simulink model "quadrotor_PID_LQR_decentralized_simulink"  (R2023b)
settings: Solver=ode4  StartTime=0.0  StopTime=10  FixedStep=0.001  RelTol=1e-3
values from neighbouring files (symbols this model uses):
  A_x_in = [0 1; 0 0]    [quadrotor_PID_Hinf_Backstepping_decentralized.m]    (also in quadrotor_PID_Hinf_Synthesis_decentralized.m; quadrotor_PID_LQR_decentralized.m)
  A_x_out = [0 1; 0 0]    [quadrotor_PID_Hinf_Backstepping_decentralized.m]    (also in quadrotor_PID_Hinf_Synthesis_decentralized.m; quadrotor_PID_LQR_decentralized.m)
  A_x_pitch = [0 1  0  0 ... (first row only)    [quadrotor_PID_LQR_decentralized.m]
  A_y_in = [0 1; 0 0]    [quadrotor_PID_Hinf_Backstepping_decentralized.m]    (also in quadrotor_PID_Hinf_Synthesis_decentralized.m; quadrotor_PID_LQR_decentralized.m)
  A_y_out = [0 1; 0 0]    [quadrotor_PID_Hinf_Backstepping_decentralized.m]    (also in quadrotor_PID_Hinf_Synthesis_decentralized.m; quadrotor_PID_LQR_decentralized.m)
  A_y_roll = [0 1  0  0 ... (first row only)    [quadrotor_PID_LQR_decentralized.m]
  Ayaw = [0 1; 0 0]    [quadrotor_PID_Hinf_Backstepping_decentralized.m]    (also in quadrotor_PID_Hinf_Synthesis_decentralized.m; quadrotor_PID_LQR_decentralized.m)
  Az = [0 1; 0 0]    [quadrotor_PID_Hinf_Backstepping_decentralized.m]    (also in quadrotor_PID_Hinf_Synthesis_decentralized.m; quadrotor_PID_LQR_decentralized.m)
  B_x_in = [0; 1/Iy]    [quadrotor_PID_Hinf_Backstepping_decentralized.m]    (also in quadrotor_PID_Hinf_Synthesis_decentralized.m; quadrotor_PID_LQR_decentralized.m)
  B_x_out = [0; g]    [quadrotor_PID_Hinf_Backstepping_decentralized.m]    (also in quadrotor_PID_Hinf_Synthesis_decentralized.m; quadrotor_PID_LQR_decentralized.m)
  B_x_pitch = [0; 0; 0; 1/Iy]    [quadrotor_PID_LQR_decentralized.m]
  B_y_in = [0; 1/Ix]    [quadrotor_PID_Hinf_Backstepping_decentralized.m]    (also in quadrotor_PID_Hinf_Synthesis_decentralized.m; quadrotor_PID_LQR_decentralized.m)
  B_y_out = [0; -g]    [quadrotor_PID_Hinf_Backstepping_decentralized.m]    (also in quadrotor_PID_Hinf_Synthesis_decentralized.m; quadrotor_PID_LQR_decentralized.m)
  B_y_roll = [0; 0; 0; 1/Ix]    [quadrotor_PID_LQR_decentralized.m]
  Byaw = [0; 1/Iz]    [quadrotor_PID_Hinf_Backstepping_decentralized.m]    (also in quadrotor_PID_Hinf_Synthesis_decentralized.m; quadrotor_PID_LQR_decentralized.m)
  Bz = [0; 1/m]    [quadrotor_PID_Hinf_Backstepping_decentralized.m]    (also in quadrotor_PID_Hinf_Synthesis_decentralized.m; quadrotor_PID_LQR_decentralized.m)
  C_x_in = [1 0]    [quadrotor_PID_Hinf_Backstepping_decentralized.m]    (also in quadrotor_PID_Hinf_Synthesis_decentralized.m; quadrotor_PID_LQR_decentralized.m)
  C_x_out = [1 0]    [quadrotor_PID_Hinf_Backstepping_decentralized.m]    (also in quadrotor_PID_Hinf_Synthesis_decentralized.m; quadrotor_PID_LQR_decentralized.m)
  C_x_pitch = [1 0 0 0]    [quadrotor_PID_LQR_decentralized.m]
  C_y_in = [1 0]    [quadrotor_PID_Hinf_Backstepping_decentralized.m]    (also in quadrotor_PID_Hinf_Synthesis_decentralized.m; quadrotor_PID_LQR_decentralized.m)
  C_y_out = [1 0]    [quadrotor_PID_Hinf_Backstepping_decentralized.m]    (also in quadrotor_PID_Hinf_Synthesis_decentralized.m; quadrotor_PID_LQR_decentralized.m)
  C_y_roll = [1 0 0 0]    [quadrotor_PID_LQR_decentralized.m]
  Cyaw = [1 0]    [quadrotor_PID_Hinf_Backstepping_decentralized.m]    (also in quadrotor_PID_Hinf_Synthesis_decentralized.m; quadrotor_PID_LQR_decentralized.m)
  Cz = [1 0]    [quadrotor_PID_Hinf_Backstepping_decentralized.m]    (also in quadrotor_PID_Hinf_Synthesis_decentralized.m; quadrotor_PID_LQR_decentralized.m)
  Ku_x_pitch = K_opt_x(5)    [quadrotor_PID_LQR_decentralized.m]
  Ku_y_roll = K_opt(5)    [quadrotor_PID_LQR_decentralized.m]
  Kx_x_pitch = K_opt_x(1:4)    [quadrotor_PID_LQR_decentralized.m]
  Kx_y_roll = K_opt(1:4)    [quadrotor_PID_LQR_decentralized.m]
undefined symbols (not defined in the file or in its folder): Kd_x_in, Kd_x_out, Kd_y_in, Kd_y_out, Kd_yaw, Kd_z, Ki_x_in, Ki_x_out, Ki_y_in, Ki_y_out, Ki_yaw, Ki_z, Kp_x_in, Kp_x_out, Kp_y_in, Kp_y_out, Kp_yaw, Kp_z, Ku_yaw, Ku_z, Kx_yaw, Kx_z
libraries: dspsrcs4 x4
settings Model: Creator=izmah  LastModifiedBy=izmah

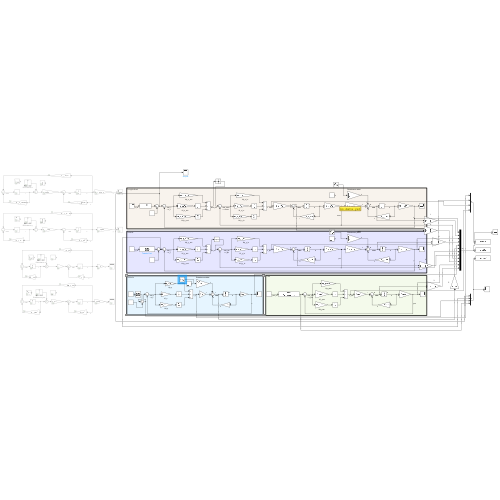
[thumbnail: Simulink's stored preview of the top-level diagram]
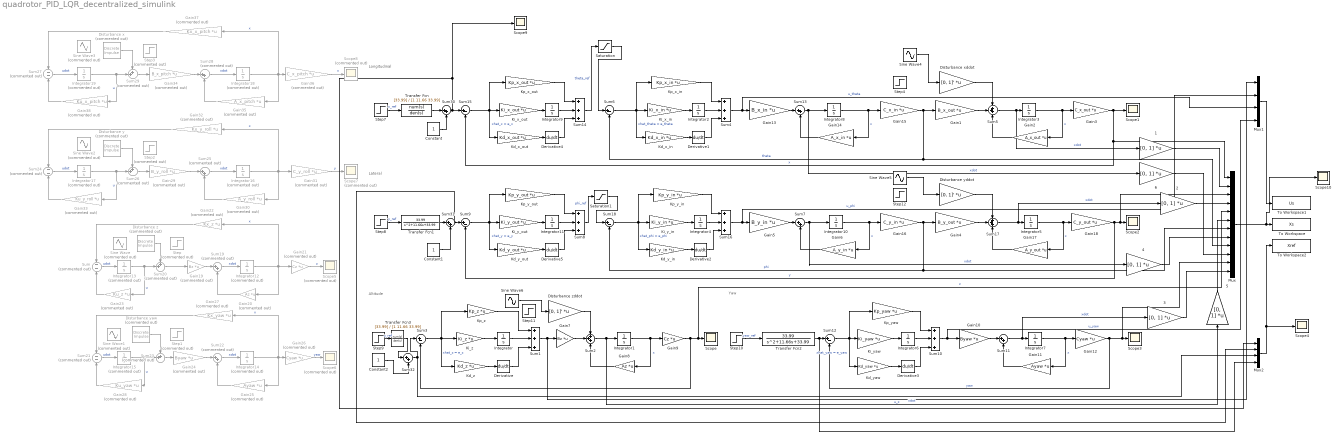
== system quadrotor_PID_LQR_decentralized_simulink ==
  note: Longitudinal
  note: Lateral
  note: Yaw
  note: Altitude
  {1..6} (6 alike) : Gain  Gain=[0, 1]  Multiplication=Matrix(K*u)
  Constant : Constant
  Constant1 : Constant
  Constant2 : Constant
  DIsturbance yddot : Gain  Gain=[0, 1]'  Multiplication=Matrix(K*u)
  DIsturbance zddot : Gain  Gain=[0, 1]'  Multiplication=Matrix(K*u)
  Derivative{,1..5} (6 alike) : Derivative
  Disturbance x : dspsrcs4/Discrete  Impulse  Commented=on  Delay=10  SampleTime=1  FrameSample=1  OutputFrames=off  dataType=double  isSigned=on  wordLen=16  udDataType=sfix(16)  fracBitsMode=Best precision  numFracBits=15  OutDataTypeStr=double  LastOutDataTypeStr=double
  Disturbance xddot : Gain  Gain=[0, 1]'  Multiplication=Matrix(K*u)
  Disturbance y : dspsrcs4/Discrete  Impulse  Commented=on  Delay=10  SampleTime=1  FrameSample=1  OutputFrames=off  dataType=double  isSigned=on  wordLen=16  udDataType=sfix(16)  fracBitsMode=Best precision  numFracBits=15  OutDataTypeStr=double  LastOutDataTypeStr=double
  Disturbance yaw : dspsrcs4/Discrete  Impulse  Commented=on  Delay=10  SampleTime=1  FrameSample=1  OutputFrames=off  dataType=double  isSigned=on  wordLen=16  udDataType=sfix(16)  fracBitsMode=Best precision  numFracBits=15  OutDataTypeStr=double  LastOutDataTypeStr=double
  Disturbance z : dspsrcs4/Discrete  Impulse  Commented=on  Delay=10  SampleTime=1  FrameSample=1  OutputFrames=off  dataType=double  isSigned=on  wordLen=16  udDataType=sfix(16)  fracBitsMode=Best precision  numFracBits=15  OutDataTypeStr=double  LastOutDataTypeStr=double
  Gain1 : Gain  Gain=B_x_out  Multiplication=Matrix(K*u)
  Gain10 : Gain  Gain=Byaw  Multiplication=Matrix(K*u)
  Gain11 : Gain  Gain=Ayaw  Multiplication=Matrix(K*u)
  Gain12 : Gain  Gain=Cyaw  Multiplication=Matrix(K*u)
  Gain13 : Gain  Gain=B_x_in  Multiplication=Matrix(K*u)
  Gain14 : Gain  Gain=A_x_in  Multiplication=Matrix(K*u)
  Gain15 : Gain  Gain=C_x_in  Multiplication=Matrix(K*u)
  Gain16 : Gain  Gain=C_y_in  Multiplication=Matrix(K*u)
  Gain17 : Gain  Gain=A_y_out  Multiplication=Matrix(K*u)
  Gain18 : Gain  Gain=C_y_out  Multiplication=Matrix(K*u)
  Gain19 : Gain  Commented=on  Gain=Bz  Multiplication=Matrix(K*u)
  Gain2 : Gain  Gain=A_x_out  Multiplication=Matrix(K*u)
  Gain20 : Gain  Commented=on  Gain=Az  Multiplication=Matrix(K*u)
  Gain21 : Gain  Commented=on  Gain=Cz  Multiplication=Matrix(K*u)
  Gain22 : Gain  Commented=on  Gain=Kx_z  Multiplication=Matrix(K*u)
  Gain23 : Gain  Commented=on  Gain=Ku_z  Multiplication=Matrix(K*u)
  Gain24 : Gain  Commented=on  Gain=Byaw  Multiplication=Matrix(K*u)
  Gain25 : Gain  Commented=on  Gain=Ayaw  Multiplication=Matrix(K*u)
  Gain26 : Gain  Commented=on  Gain=Cyaw  Multiplication=Matrix(K*u)
  Gain27 : Gain  Commented=on  Gain=Kx_yaw  Multiplication=Matrix(K*u)
  Gain28 : Gain  Commented=on  Gain=Ku_yaw  Multiplication=Matrix(K*u)
  Gain29 : Gain  Commented=on  Gain=B_y_roll  Multiplication=Matrix(K*u)
  Gain3 : Gain  Gain=C_x_out  Multiplication=Matrix(K*u)
  Gain30 : Gain  Commented=on  Gain=A_y_roll  Multiplication=Matrix(K*u)
  Gain31 : Gain  Commented=on  Gain=C_y_roll  Multiplication=Matrix(K*u)
  Gain32 : Gain  Commented=on  Gain=Kx_y_roll  Multiplication=Matrix(K*u)
  Gain33 : Gain  Commented=on  Gain=Ku_y_roll  Multiplication=Matrix(K*u)
  Gain34 : Gain  Commented=on  Gain=B_x_pitch  Multiplication=Matrix(K*u)
  Gain35 : Gain  Commented=on  Gain=A_x_pitch  Multiplication=Matrix(K*u)
  Gain36 : Gain  Commented=on  Gain=C_x_pitch  Multiplication=Matrix(K*u)
  Gain37 : Gain  Commented=on  Gain=Kx_x_pitch  Multiplication=Matrix(K*u)
  Gain38 : Gain  Commented=on  Gain=Ku_x_pitch  Multiplication=Matrix(K*u)
  Gain4 : Gain  Gain=B_y_out  Multiplication=Matrix(K*u)
  Gain5 : Gain  Gain=B_y_in  Multiplication=Matrix(K*u)
  Gain6 : Gain  Gain=A_y_in  Multiplication=Matrix(K*u)
  Gain7 : Gain  Gain=Bz  Multiplication=Matrix(K*u)
  Gain8 : Gain  Gain=Az  Multiplication=Matrix(K*u)
  Gain9 : Gain  Gain=Cz  Multiplication=Matrix(K*u)
  Integrator{,2,4,6..7,9,11} (7 alike) : Integrator
  Integrator1 : Integrator  InitialCondition=[1;0]
  Integrator10 : Integrator  InitialCondition=[0.01;0]
  Integrator{12..19} (8 alike) : Integrator  Commented=on
  Integrator3 : Integrator  InitialCondition=[1;0]
  Integrator5 : Integrator  InitialCondition=[1;0]
  Integrator8 : Integrator  InitialCondition=[0.01;0]
  Kd_x_in : Gain  Gain=Kd_x_in  Multiplication=Matrix(K*u)
  Kd_x_out : Gain  Gain=Kd_x_out  Multiplication=Matrix(K*u)
  Kd_y_in : Gain  Gain=Kd_y_in  Multiplication=Matrix(K*u)
  Kd_y_out : Gain  Gain=Kd_y_out  Multiplication=Matrix(K*u)
  Kd_yaw : Gain  Gain=Kd_yaw  Multiplication=Matrix(K*u)
  Kd_z : Gain  Gain=Kd_z  Multiplication=Matrix(K*u)
  Ki_x_in : Gain  Gain=Ki_x_in  Multiplication=Matrix(K*u)
  Ki_x_out : Gain  Gain=Ki_x_out  Multiplication=Matrix(K*u)
  Ki_y_in : Gain  Gain=Ki_y_in  Multiplication=Matrix(K*u)
  Ki_y_out : Gain  Gain=Ki_y_out  Multiplication=Matrix(K*u)
  Ki_yaw : Gain  Gain=Ki_yaw  Multiplication=Matrix(K*u)
  Ki_z : Gain  Gain=Ki_z  Multiplication=Matrix(K*u)
  Kp_x_in : Gain  Gain=Kp_x_in  Multiplication=Matrix(K*u)
  Kp_x_out : Gain  Gain=Kp_x_out  Multiplication=Matrix(K*u)
  Kp_y_in : Gain  Gain=Kp_y_in  Multiplication=Matrix(K*u)
  Kp_y_out : Gain  Gain=Kp_y_out  Multiplication=Matrix(K*u)
  Kp_yaw : Gain  Gain=Kp_yaw  Multiplication=Matrix(K*u)
  Kp_z : Gain  Gain=Kp_z  Multiplication=Matrix(K*u)
  Mux : Mux  Inputs=12
  Mux1 : Mux
  Mux2 : Mux
  Saturation : Saturate  UpperLimit=deg2rad(15)  LowerLimit=-deg2rad(15)  ZeroCross=off
  Saturation1 : Saturate  UpperLimit=deg2rad(15)  LowerLimit=-deg2rad(15)  ZeroCross=off
  Scope{,1..4,9..10} (7 alike) : Scope
  Scope{5..8} (4 alike) : Scope  Commented=on
  Sine Wave{,1..3} (4 alike) : Sin  Commented=on  SampleTime=0
  Sine Wave4 : Sin  Amplitude=5  Frequency=5  SampleTime=0
  Sine Wave5 : Sin  Amplitude=5  Frequency=5  SampleTime=0
  Sine Wave6 : Sin  Amplitude=5  Frequency=5  SampleTime=0
  Step{,1..3} (4 alike) : Step  Commented=on  Time=0  SampleTime=0
  Step10 : Step  Time=0.001  After=deg2rad(10)  SampleTime=0
  Step11 : Step  Time=0  Before=1  SampleTime=0
  Step12 : Step  Time=0  Before=1  SampleTime=0
  Step4 : Step  Time=0  Before=1  SampleTime=0
  Step7 : Step  Time=0.01  SampleTime=0
  Step8 : Step  Time=0.01  SampleTime=0
  Step9 : Step  Time=0.001  SampleTime=0
  Sum{,21,24,27} (4 alike) : Sum  Commented=on  Inputs=-|-
  Sum{1..2,4..5,8,10,14,16..17} (9 alike) : Sum  Inputs=+++
  Sum{7,11,13,30..32} (6 alike) : Sum  Inputs=|++
  Sum{3,6,9,12,15,18} (6 alike) : Sum  Inputs=|+-
  Sum{19,22,25,28} (4 alike) : Sum  Commented=on  Inputs=|++
  Sum{20,23,26,29} (4 alike) : Sum  Commented=on  Inputs=++|
  To Workspace : ToWorkspace  VariableName=Xs  SampleTime=-1
  To Workspace1 : ToWorkspace  VariableName=Us  SampleTime=-1
  To Workspace2 : ToWorkspace  VariableName=Xref  SampleTime=-1
  Transfer Fcn{,1..3} (4 alike) : TransferFcn  Numerator=[33.99]  Denominator=[1 11.66 33.99]
  wires:
  Disturbance x/1 -> Sum29/1
  Gain20/1 -> Sum19/2
  Sum28/1 -> Integrator18/1  "xdot"
  Gain22/1 -> Sum/1
  Sum20/1 -> Gain19/1
  Sum23/1 -> Gain24/1
  Sum24/1 -> Integrator17/1  "udot"
  Gain31/1 -> Scope7/1  "y"
  Gain29/1 -> Sum25/1
  Gain19/1 -> Sum19/1
  Integrator5/1 -> Gain18/1, Gain17/1  "x"
  Derivative2/1 -> Sum16/3
  Integrator17/1 -> Gain33/1, Sum26/2  "u"
  Sum27/1 -> Integrator19/1  "udot"
  Gain30/1 -> Sum25/2
  Derivative3/1 -> Sum10/3
  Gain34/1 -> Sum28/1
  Gain12/1 -> Mux/11, Scope3/1, Sum12/2  "yaw"
  Kp_y_out/1 -> Sum8/1
  Gain38/1 -> Sum27/2
  Integrator2/1 -> Sum4/2
  Gain27/1 -> Sum21/1
  Gain35/1 -> Sum28/2
  Gain26/1 -> Scope6/1  "yaw"
  Ki_y_out/1 -> Integrator11/1
  Sum21/1 -> Integrator15/1  "udot"
  Gain28/1 -> Sum21/2
  Integrator1/1 -> Gain9/1, Gain8/1  "x"
  Gain33/1 -> Sum24/2
  Disturbance y/1 -> Sum26/1
  Sum26/1 -> Gain29/1
  Gain32/1 -> Sum24/1
  Sum16/1 -> Mux1/2, Gain5/1  "u_phi"
  Gain36/1 -> Scope8/1  "x"
  Integrator19/1 -> Gain38/1, Sum29/2  "u"
  Integrator4/1 -> Sum16/2
  Sum25/1 -> Integrator16/1  "xdot"
  Disturbance yaw/1 -> Sum23/1
  Ki_yaw/1 -> Integrator6/1
  Gain3/1 -> Sum15/2, Mux/1, Scope1/1  "x"
  Integrator14/1 -> Gain26/1, Gain27/1, Gain25/1  "x"
  Sum22/1 -> Integrator14/1  "xdot"
  Gain15/1 -> Gain1/1, Mux/9, Sum6/2  "theta"
  Gain25/1 -> Sum22/2
  Integrator16/1 -> Gain32/1, Gain30/1, Gain31/1  "x"
  Gain24/1 -> Sum22/1
  Disturbance z/1 -> Sum20/1
  Integrator12/1 -> Gain22/1, Gain20/1, Gain21/1  "x"
  Sum6/1 -> Ki_x_in/1, Kp_x_in/1, Kd_x_in/1  "xhat_theta = e_theta"
  Integrator15/1 -> Gain28/1, Sum23/2  "u"
  Sum2/1 -> 5/1, Integrator1/1  "xdot"
  Gain21/1 -> Scope5/1  "z"
  Derivative/1 -> Sum1/3
  Sum3/1 -> Kd_z/1, Ki_z/1, Kp_z/1  "xhat_z = e_z"
  Gain37/1 -> Sum27/1
  Kd_y_in/1 -> Derivative2/1
  Sum18/1 -> Kd_y_in/1, Ki_y_in/1, Kp_y_in/1  "xhat_phi = e_phi"
  Sum/1 -> Integrator13/1  "udot"
  Gain23/1 -> Sum/2
  Kd_y_out/1 -> Derivative5/1
  Sum4/1 -> Mux1/3, Gain13/1  "u_theta"
  Kp_z/1 -> Sum1/1
  Ki_y_in/1 -> Integrator4/1
  Kp_x_out/1 -> Sum14/1
  Gain16/1 -> Gain4/1, Sum18/2, Mux/7  "phi"
  Gain18/1 -> Mux/3, Scope2/1, Sum9/2  "y"
  Sum12/1 -> Ki_yaw/1, Kd_yaw/1, Kp_yaw/1  "xhat_yaw = e_yaw"
  Integrator10/1 -> Gain16/1, Gain6/1  "x"
  Sum10/1 -> Mux1/4, Gain10/1  "u_yaw"
  Derivative5/1 -> Sum8/3
  Gain6/1 -> Sum7/2
  Gain5/1 -> Sum7/1
  Gain14/1 -> Sum13/2
  Kd_x_out/1 -> Derivative4/1
  Sum11/1 -> 3/1, Integrator7/1  "xdot"
  Integrator9/1 -> Sum14/2
  Gain11/1 -> Sum11/2
  Integrator11/1 -> Sum8/2
  Sum13/1 -> Integrator8/1, 6/1  "xdot"
  Integrator13/1 -> Gain23/1, Sum20/2  "u"
  Integrator6/1 -> Sum10/2
  Kp_yaw/1 -> Sum10/1
  Gain10/1 -> Sum11/1
  Integrator8/1 -> Gain14/1, Gain15/1  "x"
  Sum19/1 -> Integrator12/1  "xdot"
  Ki_x_out/1 -> Integrator9/1
  Sum15/1 -> Ki_x_out/1, Kp_x_out/1, Kd_x_out/1  "xhat_x = e_x"
  Kp_x_in/1 -> Sum4/1
  Sum7/1 -> Integrator10/1, 4/1  "xdot"
  Derivative1/1 -> Sum4/3
  Ki_z/1 -> Integrator/1
  Kd_x_in/1 -> Derivative1/1
  Sum5/1 -> 1/1, Integrator3/1  "xdot"
  Integrator7/1 -> Gain11/1, Gain12/1  "x"
  Kd_yaw/1 -> Derivative3/1
  Kp_y_in/1 -> Sum16/1
  Integrator3/1 -> Gain3/1, Gain2/1  "x"
  Ki_x_in/1 -> Integrator2/1
  Kd_z/1 -> Derivative/1
  Derivative4/1 -> Sum14/3
  Integrator/1 -> Sum1/2
  Sum17/1 -> 2/1, Integrator5/1  "xdot"
  Gain13/1 -> Sum13/1
  Sum9/1 -> Kd_y_out/1, Ki_y_out/1, Kp_y_out/1  "xhat_y = e_y"
  Integrator18/1 -> Gain37/1, Gain35/1, Gain36/1  "x"
  Sum1/1 -> Mux1/1, Gain7/1  "u_z"
  Step7/1 -> Transfer Fcn/1  "x_ref"
  Gain9/1 -> Mux/5, Scope/1, Sum3/2  "z"
  Sum29/1 -> Gain34/1
  Gain1/1 -> Sum5/2
  Gain2/1 -> Sum5/3
  DIsturbance yddot/1 -> Sum17/1
  Gain17/1 -> Sum17/3
  Gain4/1 -> Sum17/2
  Step9/1 -> Transfer Fcn3/1  "z_ref"
  DIsturbance zddot/1 -> Sum2/1
  Gain7/1 -> Sum2/2
  Gain8/1 -> Sum2/3
  Step10/1 -> Transfer Fcn2/1  "yaw_ref"
  Disturbance xddot/1 -> Sum5/1
  Step8/1 -> Transfer Fcn1/1  "y_ref"
  Transfer Fcn2/1 -> Mux2/4, Sum12/1
  Mux/1 -> Scope10/1, To Workspace/1
  Mux1/1 -> To Workspace1/1
  Transfer Fcn/1 -> Sum30/1
  Sum30/1 -> Sum15/1, Scope9/1, Mux2/1
  Constant/1 -> Sum30/2
  Transfer Fcn1/1 -> Sum31/1
  Sum31/1 -> Mux2/2, Sum9/1
  Constant1/1 -> Sum31/2
  Transfer Fcn3/1 -> Sum32/1
  Sum32/1 -> Mux2/3, Sum3/1
  Constant2/1 -> Sum32/2
  Mux2/1 -> To Workspace2/1, Scope4/1
  1/1 -> Mux/2
  2/1 -> Mux/4
  3/1 -> Mux/12
  4/1 -> Mux/8
  5/1 -> Mux/6
  6/1 -> Mux/10
  Sum14/1 -> Saturation/1  "theta_ref"
  Saturation/1 -> Sum6/1
  Sum8/1 -> Saturation1/1  "phi_ref"
  Saturation1/1 -> Sum18/1
  Sine Wave4/1 -> Disturbance xddot/1
  Sine Wave6/1 -> DIsturbance zddot/1
  Sine Wave5/1 -> DIsturbance yddot/1
